simulink model "SimulationGuidedRecoveryV2"  (R2024b)
settings: Solver=VariableStepAuto  StartTime=0.0  StopTime=1500  RelTol=1e-3
libraries: aerolibwind2 x1, slpidlib x1
settings Model: Creator=Jerry Gao  LastModifiedBy=bgbg0
settings RTWCC: GPUComputeCapability=3.5

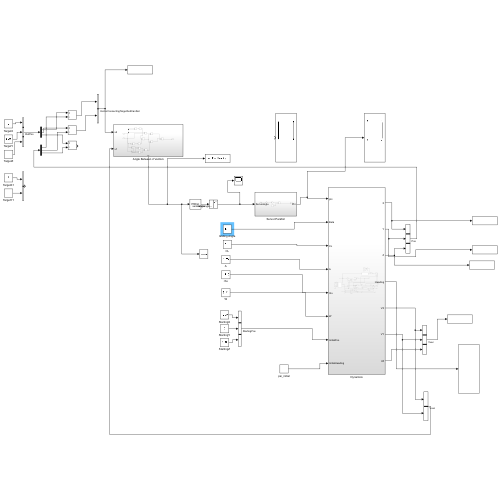
[thumbnail: Simulink's stored preview of the top-level diagram]
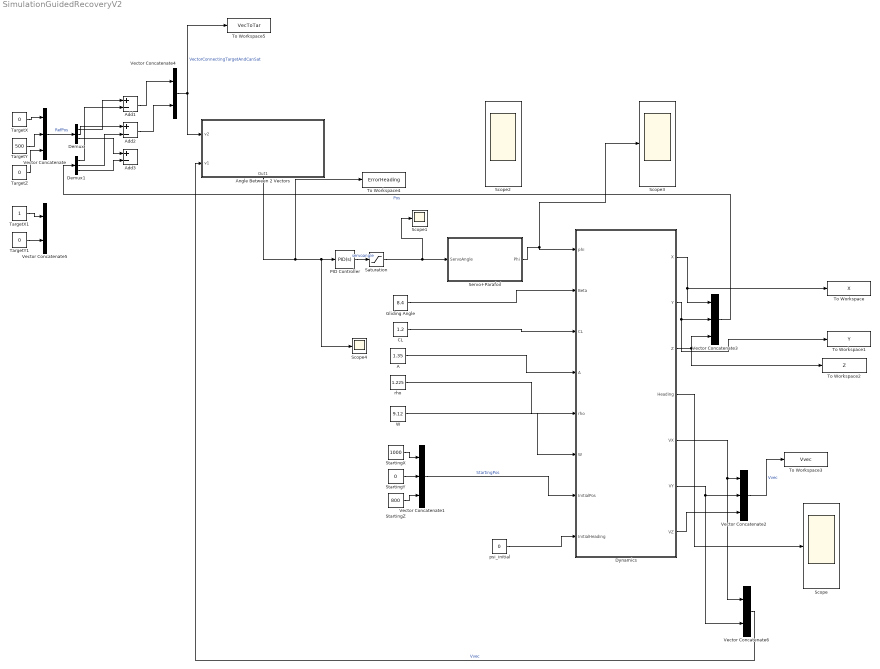
== system SimulationGuidedRecoveryV2 ==
  A : Constant  Value=1.35
  Add1 : Sum  Inputs=+-
  Add2 : Sum  Inputs=+-
  Add3 : Sum  Inputs=+-
  Angle Between 2 Vectors : Subsystem
      settings: PortSchema="{\"entries\":[{\"content\":{\"sides\":[{\"content\":{\"connectorIds\":[\"In1\",\"In2\"]},\"type\":\"ConnectorPlacement.EquallySpacedRectSide\",\"uuid\":\"2a3f35bb-975b-4170-bf2f-b66643bf7732\"},{\"content\":{\"side\":\"RIGHT\"},\"type\":\"ConnectorPlacement.EquallySpacedRectSide\",\"uuid\":\"e83cc06c-abd1-4e89-a0f4-1a246757fc80\"},{\"content\":{\"side\":\"TOP\"},\"type\":\"ConnectorPlacement.EquallySpacedRectSide\",\"uuid\":\"eeba1ec8-f966-4d1c-ad11-91f5f0644dce\"},{\"content\":{\"connectorIds\":[\"Out1\"],\"side\":\"BOTTOM\"},\"type\":\"ConnectorPlacement.EquallySpacedRectSide\",\"uuid\":\"aaaa25ac-3a4f-40f7-9fcb-849203176940\"}]},\"type\":\"ConnectorPlacement.EquallySpacedConnector\",\"uuid\":\"d0b184af-993a-4781-b8c0-335e8ad5db02\"}],\"packageUris\":[\"http://schema.mathworks.com/mf0/Connector/R2020b\"],\"version\":\"1.0\"}"
  CL : Constant  Value=1.2
  Demux : Demux  Outputs=3
  Demux1 : Demux  Outputs=3
  Dynamics : Subsystem
  Gliding Angle : Constant  Value=8.4
  PID Controller : slpidlib/PID Controller  Controller=PID  Form=Parallel  TimeDomain=Continuous-time  UseExternalTs=off  SampleTime=-1  IntegratorMethod=Forward Euler  FilterMethod=Forward Euler  ControllerParametersSource=internal  P=144.769965332485  I=1.05397863888132  UseKiTs=off  D=-31.9542651869893  UseExternalDerivativeSource=off  N=4.53053651790529  UseFilter=on  TunerSelectOption=Transfer Function Based (PID Tuner App)  InitialConditionSource=internal  InitialConditionForIntegrator=0  InitialConditionForFilter=0  DifferentiatorICPrevScaledInput=0  ExternalReset=none  TrackingMode=off  Kt=1  LimitOutput=off  SatLimitsSource=internal  UpperSaturationLimit=inf  LowerSaturationLimit=-inf  LinearizeAsGain=on  AntiWindupMode=none  Kb=1  LimitIntegrator=off  UpperIntegratorSaturationLimit=inf  LowerIntegratorSaturationLimit=-inf  POutMin=[]  POutMax=[]  IOutMin=[]  IOutMax=[]  DOutMin=[]  DOutMax=[]  NOutMin=[]  NOutMax=[]  SumOutMin=[]  SumOutMax=[]  SaturationOutMin=[]  SaturationOutMax=[]  PParamMin=[]  PParamMax=[]  IParamMin=[]  IParamMax=[]  DParamMin=[]  DParamMax=[]  NParamMin=[]  NParamMax=[]  KbParamMin=[]  KbParamMax=[]  KtParamMin=[]  KtParamMax=[]  KbOutMin=[]  KbOutMax=[]  KtOutMin=[]  KtOutMax=[]  IntegratorOutMin=[]  IntegratorOutMax=[]  FilterOutMin=[]  FilterOutMax=[]  SumI1OutMin=[]  SumI1OutMax=[]  SumI2OutMin=[]  SumI2OutMax=[]  SumI3OutMin=[]  SumI3OutMax=[]  SumI4OutMin=[]  SumI4OutMax=[]  SumDOutMin=[]  SumDOutMax=[]  DifferentiatorOutMin=[]  DifferentiatorOutMax=[]  FilterDiffOutCoefMin=[]  FilterDiffOutCoefMax=[]  ReciprocalOutMin=[]  ReciprocalOutMax=[]  SumDenOutMin=[]  SumDenOutMax=[]  SumNumOutMin=[]  SumNumOutMax=[]  DivideOutMin=[]  DivideOutMax=[]  UdiffTsProdOutMin=[]  UdiffTsProdOutMax=[]  NTsProdOutMin=[]  NTsProdOutMax=[]  UintegralTsProdOutMin=[]  UintegralTsProdOutMax=[]  UngainTsProdOutMin=[]  UngainTsProdOutMax=[]  ClampingZeroOutDataTypeStr=Inherit: Inherit via back propagation  ClampingZeroOutMin=[]  ClampingZeroOutMax=[]  FilterDenConstantOutDataTypeStr=Inherit: Inherit via back propagation  FilterDenConstantOutMin=[]  FilterDenConstantOutMax=[]  PCopyOutDataTypeStr=Inherit: Inherit via back propagation  PCopyOutMin=[]  PCopyOutMax=[]  NCopyOutDataTypeStr=Inherit: Inherit via back propagation  NCopyOutMin=[]  NCopyOutMax=[]  IntegratorContinuousStateAttributes=''  IntegratorStateMustResolveToSignalObject=off  IntegratorRTWStateStorageClass=Auto  FilterContinuousStateAttributes=''  FilterStateMustResolveToSignalObject=off  FilterRTWStateStorageClass=Auto  ParallelPVariant=InternalParameters  IdealPVariant=Disabled  IVariant=InternalParameters  DVariant=InternalParameters  IntegratorVariant=Continuous  SatVariant=Disabled  AWVariant=Passthrough  PCopyVariant=Disabled  TRVariant=Disabled  FdbkBlocksVariant=Forward  IdealPFdbkVariant=Disabled  SatFdbkVariant=Disabled  DerivativeFilterVariant=ContFilter  NVariant=InternalParameters  NCopyVariant=Disabled  FilterICVariant=InternalICsFilter  IntegratorICVariant=InternalICs  ExternalResetVariant=Disabled  TRSumVariant=Passthrough  SumFdbkVariant=Disabled  SumVariant=Sum_PID  TsampFilterVariant=InternalTs  TsampNgainVariant=Passthrough  TsampIntegralVariant=Disabled_SignalSpec  ExternalSaturationOutDataTypeStr=Inherit: Same as second input  DerivativeSourceVariant=ErrorSignal  PreIntVariant=InternalPreInt
  Saturation : Saturate  UpperLimit=1260  LowerLimit=-1260
  Scope{,1..4} (5 alike) : Scope
  Servo+Parafoil : Subsystem
  StartingX : Constant  Value=1000
  StartingY : Constant  Value=0
  StartingZ : Constant  Value=800
  TargetX : Constant  Value=0
  TargetX1 : Constant
  TargetY : Constant  Value=500
  TargetY1 : Constant  Value=0
  TargetZ : Constant  Value=0
  To Workspace : ToWorkspace  VariableName=X  SaveFormat=Timeseries  SampleTime=-1
  To Workspace1 : ToWorkspace  VariableName=Y  SaveFormat=Timeseries  SampleTime=-1
  To Workspace2 : ToWorkspace  VariableName=Z  SaveFormat=Timeseries  SampleTime=-1
  To Workspace3 : ToWorkspace  VariableName=Vvec  SaveFormat=Timeseries  SampleTime=-1
  To Workspace4 : ToWorkspace  VariableName=ErrorHeading  SaveFormat=Timeseries  SampleTime=-1
  To Workspace5 : ToWorkspace  VariableName=VecToTar  SaveFormat=Timeseries  SampleTime=-1
  Vector Concatenate{,1..3} (4 alike) : Concatenate  NumInputs=3
  Vector Concatenate4 : Concatenate
  Vector Concatenate5 : Concatenate
  Vector Concatenate6 : Concatenate
  W : Constant  Value=9.12
  psi_initial : Constant  Value=0
  rho : Constant  Value=1.225
  wires:
  Gliding Angle/1 -> Dynamics/2(Beta)
  CL/1 -> Dynamics/3(CL)
  A/1 -> Dynamics/4(A)
  rho/1 -> Dynamics/5(rho)
  W/1 -> Dynamics/6(W)
  TargetX/1 -> Vector Concatenate/1
  TargetY/1 -> Vector Concatenate/2
  StartingY/1 -> Vector Concatenate1/2
  StartingZ/1 -> Vector Concatenate1/3
  StartingX/1 -> Vector Concatenate1/1
  Vector Concatenate1/1 -> Dynamics/7(InitialPos)  "StartingPos"
  Servo+Parafoil/1(Phi) -> Scope3/1, Dynamics/1(phi)
  PID Controller/1 -> Saturation/1  "servoangle"
  psi_initial/1 -> Dynamics/8(InitialHeading)
  Dynamics/1(X) -> Vector Concatenate3/1, To Workspace/1
  Dynamics/2(Y) -> To Workspace1/1, Vector Concatenate3/2
  Vector Concatenate3/1 -> Demux1/1  "Pos"
  Dynamics/4(Heading) -> Scope/1
  Vector Concatenate/1 -> Demux/1  "RefPos"
  Demux/1 -> Add1/1
  Demux1/1 -> Add1/2
  Demux/2 -> Add2/1
  Demux1/2 -> Add2/2
  Add1/1 -> Vector Concatenate4/1
  Add2/1 -> Vector Concatenate4/2
  Dynamics/3(Z) -> To Workspace2/1, Vector Concatenate3/3
  Vector Concatenate4/1 -> Angle Between 2 Vectors/1(v2), To Workspace5/1  "VectorConnectingTargetAndCanSat"
  TargetY1/1 -> Vector Concatenate5/2
  TargetX1/1 -> Vector Concatenate5/1
  Angle Between 2 Vectors/1(Out1) -> PID Controller/1, Scope4/1, To Workspace4/1
  Dynamics/5(VX) -> Vector Concatenate6/1, Vector Concatenate2/1
  Dynamics/6(VY) -> Vector Concatenate6/2, Vector Concatenate2/2
  Dynamics/7(VZ) -> Vector Concatenate2/3
  Vector Concatenate2/1 -> To Workspace3/1  "Vvec"
  TargetZ/1 -> Vector Concatenate/3
  Demux/3 -> Add3/1
  Demux1/3 -> Add3/2
  Vector Concatenate6/1 -> Angle Between 2 Vectors/2(v1)  "Vvec"
  Saturation/1 -> Scope1/1, Servo+Parafoil/1(ServoAngle)

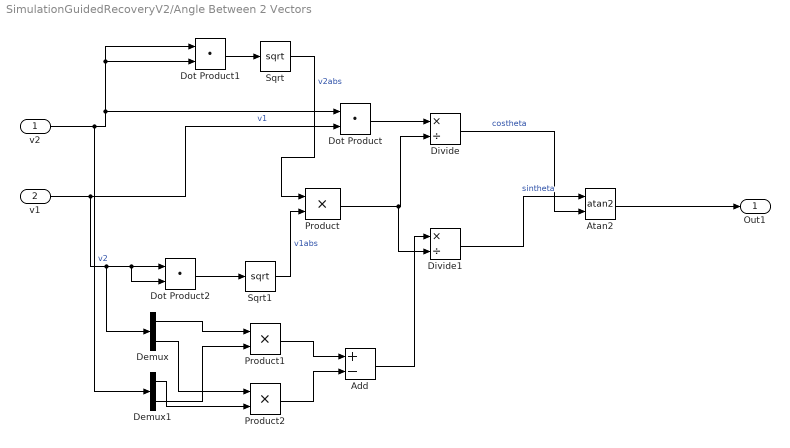
== system SimulationGuidedRecoveryV2/Angle Between 2 Vectors ==
  v2 : Inport
  v1 : Inport  Port=2
  Add : Sum  Inputs=+-
  Atan2 : Trigonometry  Operator=atan2
  Demux : Demux  Outputs=2
  Demux1 : Demux  Outputs=2
  Divide : Product  Inputs=*/
  Divide1 : Product  Inputs=*/
  Dot Product : DotProduct  OutDataTypeStr=Inherit: Inherit via internal rule
  Dot Product1 : DotProduct  OutDataTypeStr=Inherit: Inherit via internal rule
  Dot Product2 : DotProduct  OutDataTypeStr=Inherit: Inherit via internal rule
  Product : Product
  Product1 : Product
  Product2 : Product
  Sqrt : Sqrt
  Sqrt1 : Sqrt
  Out1 : Outport
  wires:
  v1/1 -> Demux/1, Dot Product2/2, Dot Product2/1, Dot Product/2  "v1"
  Dot Product1/1 -> Sqrt/1
  Dot Product2/1 -> Sqrt1/1
  Sqrt/1 -> Product/1  "v2abs"
  Sqrt1/1 -> Product/2  "v1abs"
  Dot Product/1 -> Divide/1
  Product/1 -> Divide1/2, Divide/2
  Divide/1 -> Atan2/2  "costheta"
  v2/1 -> Demux1/1, Dot Product1/2, Dot Product1/1, Dot Product/1  "v2"
  Add/1 -> Divide1/1
  Divide1/1 -> Atan2/1  "sintheta"
  Atan2/1 -> Out1/1
  Demux/1 -> Product1/1
  Demux1/2 -> Product1/2
  Demux/2 -> Product2/1
  Demux1/1 -> Product2/2
  Product1/1 -> Add/1
  Product2/1 -> Add/2

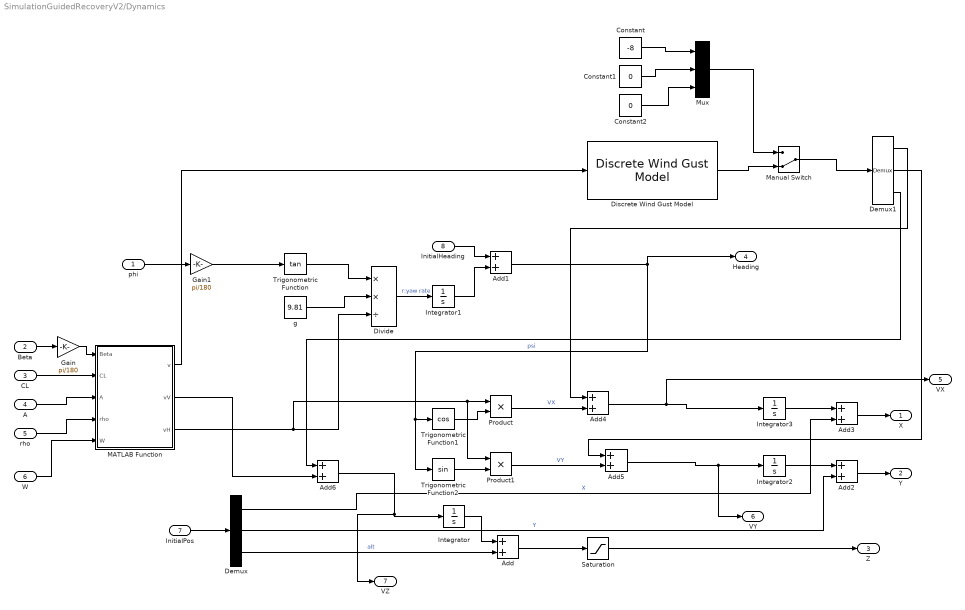
== system SimulationGuidedRecoveryV2/Dynamics ==
  phi : Inport
  Beta : Inport  Port=2
  CL : Inport  Port=3
  A : Inport  Port=4
  rho : Inport  Port=5
  W : Inport  Port=6
  InitialPos : Inport  Port=7
  InitialHeading : Inport  Port=8
  Add{,1..6} (7 alike) : Sum
  Constant : Constant  Value=-8
  Constant1 : Constant  Value=0
  Constant2 : Constant  Value=0
  Demux : Demux  Outputs=3
  Demux1 : Demux  Outputs=3
  Discrete Wind Gust Model : aerolibwind2/Discrete Wind Gust Model  units=Metric (MKS)  Gx=on  Gy=on  Gz=on  t_0=5  d_m=[100 100 50]  v_m=[1 0 0]
  Divide : Product  Inputs=**/
  Gain : Gain  Gain=pi/180
  Gain1 : Gain  Gain=pi/180
  Integrator{,1..3} (4 alike) : Integrator
  MATLAB Function : MATLAB Function  TreatAsAtomicUnit=on
  Manual Switch : ManualSwitch  CurrentSetting=0
  Mux : Mux  Inputs=3
  Product : Product
  Product1 : Product
  Saturation : Saturate  UpperLimit=1000  LowerLimit=0
  Trigonometric Function : Trigonometry  Operator=tan
  Trigonometric Function1 : Trigonometry  Operator=cos
  Trigonometric Function2 : Trigonometry
  g : Constant  Value=9.81
  X : Outport
  Y : Outport  Port=2
  Z : Outport  Port=3
  Heading : Outport  Port=4
  VX : Outport  Port=5
  VY : Outport  Port=6
  VZ : Outport  Port=7
  wires:
  Beta/1 -> Gain/1
  CL/1 -> MATLAB Function/2(CL)
  A/1 -> MATLAB Function/3(A)
  rho/1 -> MATLAB Function/4(rho)
  W/1 -> MATLAB Function/5(W)
  Gain/1 -> MATLAB Function/1(Beta)
  InitialPos/1 -> Demux/1
  Demux/3 -> Add/2  "alt"
  Demux/2 -> Add2/2  "Y"
  Demux/1 -> Add3/2  "X"
  Integrator/1 -> Add/1
  Add/1 -> Saturation/1
  phi/1 -> Gain1/1
  g/1 -> Divide/2
  Trigonometric Function/1 -> Divide/1
  Divide/1 -> Integrator1/1  "r:yaw rate"
  Integrator1/1 -> Add1/2
  InitialHeading/1 -> Add1/1
  Trigonometric Function1/1 -> Product/2
  Trigonometric Function2/1 -> Product1/2
  MATLAB Function/3(vH) -> Divide/3, Product1/1, Product/1
  Integrator3/1 -> Add3/1
  Integrator2/1 -> Add2/1
  Add2/1 -> Y/1
  Add3/1 -> X/1
  Saturation/1 -> Z/1
  Gain1/1 -> Trigonometric Function/1
  Add1/1 -> Heading/1, Trigonometric Function2/1, Trigonometric Function1/1  "psi"
  MATLAB Function/1(v) -> Discrete Wind Gust Model/1
  Product/1 -> Add4/2  "VX"
  Add4/1 -> VX/1, Integrator3/1
  Add5/1 -> VY/1, Integrator2/1
  Product1/1 -> Add5/2  "VY"
  Add6/1 -> VZ/1, Integrator/1
  MATLAB Function/2(vV) -> Add6/2
  Demux1/2 -> Add5/1
  Demux1/1 -> Add4/1
  Demux1/3 -> Add6/1
  Manual Switch/1 -> Demux1/1
  Discrete Wind Gust Model/1 -> Manual Switch/2
  Mux/1 -> Manual Switch/1
  Constant2/1 -> Mux/3
  Constant1/1 -> Mux/2
  Constant/1 -> Mux/1

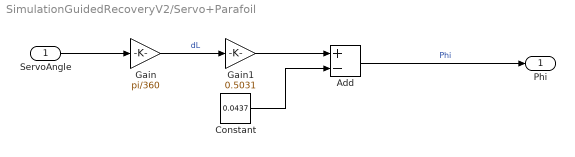
== system SimulationGuidedRecoveryV2/Servo+Parafoil ==
  ServoAngle : Inport
  Add : Sum  Inputs=+-
  Constant : Constant  Value=0.0437
  Gain : Gain  Gain=pi/360
  Gain1 : Gain  Gain=0.5031
  Phi : Outport
  wires:
  ServoAngle/1 -> Gain/1
  Gain/1 -> Gain1/1  "dL"
  Constant/1 -> Add/2
  Gain1/1 -> Add/1
  Add/1 -> Phi/1  "Phi"

== matlab function SimulationGuidedRecoveryV2/Dynamics/MATLAB Function ==
  data: Beta input; v output; CL input; A input; rho input; W input; vV output; vH output
function [v,vV,vH]= findGlidingSpeed(Beta,CL,A,rho,W)

    L = W/(cos(Beta) + tan(Beta)*sin(Beta));
    v = sqrt(2*L/(rho*A*CL));
    vV = -v*sin(Beta);
    vH = v*cos(Beta);
end
